simulink model "ChildApp"  (R2023a)
settings: Solver=FixedStepAuto  StartTime=0.0  StopTime=10  RelTol=1e-3
libraries: androidcommunicationlib x6, androiduilib x5, androidaudiovideolib x4, androidsensorlib x3
settings Model: Creator=Hitesh  LastModifiedBy=Hitesh
settings DataIOCC: SaveFormat=Array  InspectSignalLogs=on
settings OptimizationCC: EnhancedBackFolding=on  PassReuseOutputArgsAs=Individual arguments  ZeroExternalMemoryAtStartup=off  ZeroInternalMemoryAtStartup=off  MaxStackSize=64  OptimizeBlockOrder=speed  DifferentSizesBufferReuse=on  OptimizationCustomize=off  EfficientTunableParamExpr=on
settings DebuggingCC: ParameterTunabilityLossMsg=error
settings HardwareCC: ProdBitPerLong=64  ProdLargestAtomicInteger=LongLong  ProdLargestAtomicFloat=Double  ProdLongLongMode=on  ProdHWDeviceType=ARM Compatible->ARM 64-bit (LP64)
settings SFSimCC: MATLABDynamicMemAlloc=off
settings RTWCC: Description=Embedded Coder  SystemTargetFile=ert.tlc  HardwareBoard=Android Device (64bit)  TLCOptions="-aInlineSetEventsForThisBaseRateFcn=TLC_FALSE -aSuppressMultiTaskScheduler=TLC_FALSE  -aRateBasedStepFcn=0"  TemplateMakefile=ert_default_tmf  RTWVerbose=off  Toolchain=Android SDK/NDK Tools
settings CodeAppCC: ForceParamTrailComments=on  IgnoreCustomStorageClasses=off  OperatorAnnotations=on  SimulinkDataObjDesc=on  SFDataObjDesc=on  InsertBlockDesc=on

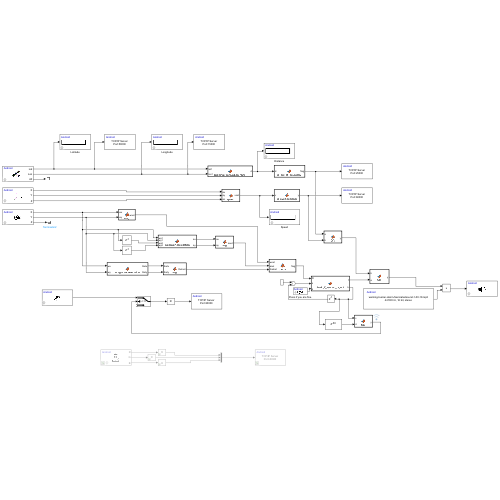
[thumbnail: Simulink's stored preview of the top-level diagram]
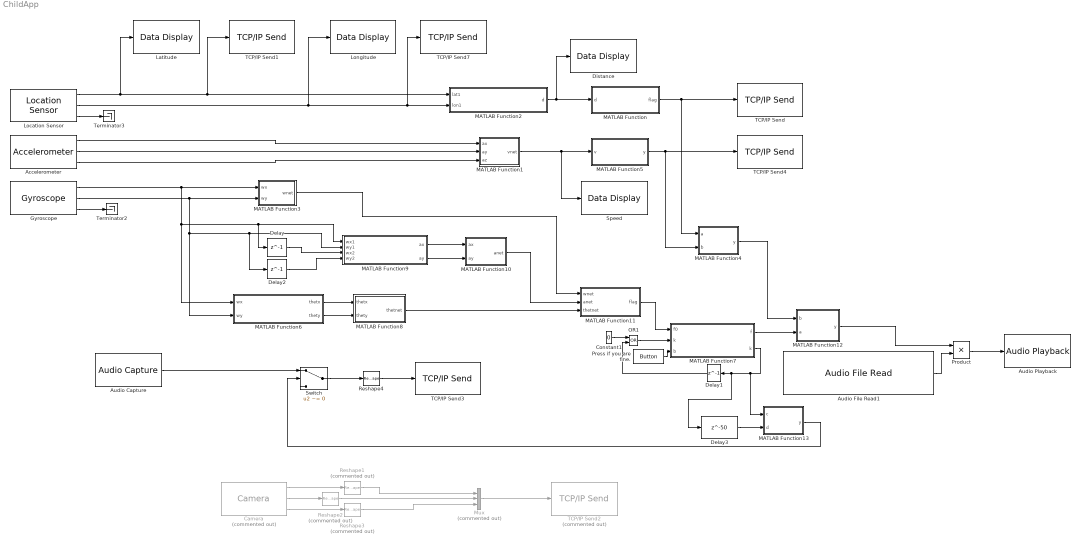
== system ChildApp ==
  Accelerometer : androidsensorlib/Accelerometer  OutputVector=off  SampleTime=0.2  BlockPlatform=Android
  Audio Capture : androidaudiovideolib/Audio Capture  SampleFreq=44100  FrameSize=4410  SampleTime=0.1  SimulateUsing=Code generation  DeviceStr=0  QueueDuration=0  BlockPlatform=Android  AudioSamplingFreq=44100
  Audio File Read1 : androidaudiovideolib/Audio File Read  FileName=C:\Users\Hitesh\Downloads\warning-buzzer-alarm-fascinatedsound-1-00-18.mp3  FrameSize=4410
  Audio Playback : androidaudiovideolib/Audio Playback  SampleFreq=44100  AudioSamplingFreq=44100  SampleTime=0.1  DeviceStr=0  QueueDuration=0  BlockPlatform=Android
  Camera : androidaudiovideolib/Camera  Commented=on  CameraLocation=Back  CameraResolutions=Back - 320x240  Width=320  Height=240  SampleTime=2  BlockPlatform=Android
  Constant1 : Constant  Value=0  OutDataTypeStr=double
  Delay : Delay  DelayLength=1
  Delay1 : Delay  DelayLength=1  InitialCondition=0
  Delay2 : Delay  DelayLength=1
  Delay3 : Delay  DelayLength=50  InitialCondition=0
  Distance : androiduilib/Data Display  DataDisplayId=ChildApp/Distance  Format=Float  Precision=6  SimulateUsing=Code generation  blockPlatform=Android
  Gyroscope : androidsensorlib/Gyroscope  OutputVector=off  SampleTime=0.2  BlockPlatform=Android
  Latitude : androiduilib/Data Display  DataDisplayId=ChildApp/Latitude  Format=Float  Precision=6  SimulateUsing=Code generation  blockPlatform=Android
  Location Sensor : androidsensorlib/Location Sensor  OutputVector=off  SampleTime=0.1  BlockPlatform=Android
  Longitude : androiduilib/Data Display  DataDisplayId=ChildApp/Longitude  Format=Float  Precision=6  SimulateUsing=Code generation  blockPlatform=Android
  MATLAB Function : MATLAB Function  TreatAsAtomicUnit=on
  MATLAB Function1 : MATLAB Function  TreatAsAtomicUnit=on
  MATLAB Function10 : MATLAB Function  TreatAsAtomicUnit=on
  MATLAB Function11 : MATLAB Function  TreatAsAtomicUnit=on
  MATLAB Function12 : MATLAB Function  TreatAsAtomicUnit=on
  MATLAB Function13 : MATLAB Function  TreatAsAtomicUnit=on
  MATLAB Function2 : MATLAB Function  TreatAsAtomicUnit=on
  MATLAB Function3 : MATLAB Function  TreatAsAtomicUnit=on
  MATLAB Function4 : MATLAB Function  TreatAsAtomicUnit=on
  MATLAB Function5 : MATLAB Function  TreatAsAtomicUnit=on
  MATLAB Function6 : MATLAB Function  TreatAsAtomicUnit=on
  MATLAB Function7 : MATLAB Function  TreatAsAtomicUnit=on
  MATLAB Function8 : MATLAB Function  TreatAsAtomicUnit=on
  MATLAB Function9 : MATLAB Function  TreatAsAtomicUnit=on
  Mux : Mux  Commented=on  Inputs=3
  OR1 : Logic  Operator=OR  IconShape=distinctive  AllPortsSameDT=off  OutDataTypeStr=boolean
  Press if you are fine. : androiduilib/Button  ButtonState=Not pressed  ButtonId=ChildApp/Press_if_you_are_fine.  State=off  SampleTime=0.1  BlockPlatform=Android
  Product : Product  InputSameDT=on  OutDataTypeStr=Inherit: Same as first input
  Reshape1 : Reshape  Commented=on  OutputDimensionality=Customize  OutputDimensions=[320*240,1]
  Reshape2 : Reshape  Commented=on  OutputDimensionality=Customize  OutputDimensions=[320*240,1]
  Reshape3 : Reshape  Commented=on  OutputDimensionality=Customize  OutputDimensions=[320*240,1]
  Reshape4 : Reshape  OutputDimensionality=Customize  OutputDimensions=[8820,1]
  Speed : androiduilib/Data Display  DataDisplayId=ChildApp/Speed  Format=Float  Precision=6  SimulateUsing=Code generation  blockPlatform=Android
  Switch : Switch  Criteria=u2 ~= 0  OutDataTypeStr=int16  SaturateOnIntegerOverflow=off  InputSameDT=off
  TCP/IP Send : androidcommunicationlib/TCP//IP Send  TCPSendId=ChildApp/TCP//IP_Send  Mode_=Server  LocalServerPort_=25000  RemoteAddr_=137.158.24.15  RemoteServerPort_=38000  ClientPortBindingSelection_=off  ClientPortToBind_=35000  BlockingMode_=off  BlockTimeout_=0.1
  TCP/IP Send1 : androidcommunicationlib/TCP//IP Send  TCPSendId=ChildApp/TCP//IP_Send1  Mode_=Server  LocalServerPort_=50000  RemoteAddr_=127.0.0.1  RemoteServerPort_=25000  ClientPortBindingSelection_=off  ClientPortToBind_=35000  BlockingMode_=off  BlockTimeout_=0.1
  TCP/IP Send2 : androidcommunicationlib/TCP//IP Send  Commented=on  TCPSendId=ChildApp/TCP//IP_Send2  Mode_=Server  LocalServerPort_=45000  RemoteAddr_=137.158.24.15  RemoteServerPort_=38000  ClientPortBindingSelection_=off  ClientPortToBind_=35000  BlockingMode_=off  BlockTimeout_=0.1
  TCP/IP Send3 : androidcommunicationlib/TCP//IP Send  TCPSendId=ChildApp/TCP//IP_Send3  Mode_=Server  LocalServerPort_=20000  RemoteAddr_=137.158.24.15  RemoteServerPort_=38000  ClientPortBindingSelection_=off  ClientPortToBind_=35000  BlockingMode_=off  BlockTimeout_=0.1
  TCP/IP Send4 : androidcommunicationlib/TCP//IP Send  TCPSendId=ChildApp/TCP//IP_Send4  Mode_=Server  LocalServerPort_=60000  RemoteAddr_=137.158.24.15  RemoteServerPort_=38000  ClientPortBindingSelection_=off  ClientPortToBind_=35000  BlockingMode_=off  BlockTimeout_=0.1
  TCP/IP Send7 : androidcommunicationlib/TCP//IP Send  TCPSendId=ChildApp/TCP//IP_Send7  Mode_=Server  LocalServerPort_=15000  RemoteAddr_=127.0.0.1  RemoteServerPort_=25000  ClientPortBindingSelection_=off  ClientPortToBind_=35000  BlockingMode_=off  BlockTimeout_=0.1
  Terminator2 : Terminator
  Terminator3 : Terminator
  wires:
  Gyroscope/1 -> MATLAB Function6/1(wx), Delay/1, MATLAB Function9/1(wx1), MATLAB Function3/1(wx)
  Gyroscope/2 -> MATLAB Function6/2(wy), Delay2/1, MATLAB Function9/2(wy1), MATLAB Function3/2(wy)
  Delay2/1 -> MATLAB Function9/4(wy2)
  Product/1 -> Audio Playback/1
  MATLAB Function3/1(wnet) -> MATLAB Function11/1(wnet)
  Delay1/1 -> OR1/2
  Delay/1 -> MATLAB Function9/3(wx2)
  MATLAB Function6/1(thetx) -> MATLAB Function8/1(thetx)
  MATLAB Function6/2(thety) -> MATLAB Function8/2(thety)
  Location Sensor/2 -> MATLAB Function2/2(lon1), TCP/IP Send7/1, Longitude/1
  Accelerometer/1 -> MATLAB Function1/1(ax)
  Accelerometer/2 -> MATLAB Function1/2(ay)
  MATLAB Function5/1(y) -> MATLAB Function4/2(b), TCP/IP Send4/1
  Accelerometer/3 -> MATLAB Function1/3(az)
  MATLAB Function9/2(ay) -> MATLAB Function10/2(ay)
  MATLAB Function9/1(ax) -> MATLAB Function10/1(ax)
  MATLAB Function8/1(thetnet) -> MATLAB Function11/3(thetnet)
  Constant1/1 -> OR1/1
  MATLAB Function2/1(d) -> MATLAB Function/1(d), Distance/1
  MATLAB Function11/1(flag) -> MATLAB Function7/1(f0)
  MATLAB Function1/1(vnet) -> Speed/1, MATLAB Function5/1(v)
  MATLAB Function10/1(anet) -> MATLAB Function11/2(anet)
  Press if you are fine./1 -> MATLAB Function7/3(b)
  OR1/1 -> MATLAB Function7/2("k ")
  MATLAB Function7/1(f) -> MATLAB Function12/2(a)
  MATLAB Function/1(flag) -> MATLAB Function4/1(a), TCP/IP Send/1
  MATLAB Function4/1(y) -> MATLAB Function12/1(b)
  MATLAB Function12/1(y) -> Product/1
  Audio File Read1/1 -> Product/2
  Gyroscope/3 -> Terminator2/1
  Location Sensor/3 -> Terminator3/1
  Audio Capture/1 -> Switch/1
  Switch/1 -> Reshape4/1
  Camera/1 -> Reshape1/1
  Camera/3 -> Reshape3/1
  Camera/2 -> Reshape2/1
  Reshape4/1 -> TCP/IP Send3/1
  Mux/1 -> TCP/IP Send2/1
  Reshape1/1 -> Mux/1
  Reshape2/1 -> Mux/2
  Reshape3/1 -> Mux/3
  Delay3/1 -> MATLAB Function13/2(d)
  MATLAB Function13/1(y) -> Switch/2
  MATLAB Function7/2(k) -> MATLAB Function13/1(c), Delay3/1, Delay1/1
  Location Sensor/1 -> MATLAB Function2/1(lat1), TCP/IP Send1/1, Latitude/1

== matlab function ChildApp/MATLAB Function8 ==
  data: thetx input; thetnet output; thety input
function thetnet = mag(thetx,thety)
    thetnet = sqrt(thetx^2+thety^2);
end

== matlab function ChildApp/MATLAB Function9 ==
  data: wx1 input; ax output; wy1 input; wx2 input; wy2 input; ay output
function [ax,ay] = integrateAcceleration(wx1,wy1,wx2,wy2)
    dt=0.2;
    ax=(wx2-wx1)/dt;
    ay=(wy2-wy1)/dt;
end

== matlab function ChildApp/MATLAB Function12 ==
  data: b input; y output; a input
function y = OR(b,a)
    if(b == 1 || a == 1)
        y = int16(1);
    else
        y = int16(0);
    end
end

== matlab function ChildApp/MATLAB Function13 ==
  data: c input; d input; y output
function y = fcn(c,d)
    if(c == 1)
        if(d == 1)
            y = int16(1);
        else
            y = int16(0);
        end
    else
        y = int16(0);
    end
end

== matlab function ChildApp/MATLAB Function1 ==
  data: ax input; vnet output; ay input; az input
function vnet = speed(ax,ay,az)
    dt = 0.2;
    vx = double(ax)*dt;
    vy = double(ay)*dt;
    vz = double(az-9.81)*dt;
    vnet = sqrt(vx^2+vy^2+vz^2);
    if( vnet<= 0.2)
        vnet = 0;
    end
end

== matlab function ChildApp/MATLAB Function2 ==
  data: lat1 input; d output; lon1 input
function d = DistanceFromLatLonInKm(lat1,lon1)
    R = 6371;
    lat2 = 23.2096737;
    lon2 = 72.6836191;
    % Haversine formula
    dlat = deg2rad(lat2-lat1);
    dlon = deg2rad(lon2-lon1); 
    a = sin(dlat/2)^2 + cos(lat1)* cos(lat2) * sin(dlon/2)^2;
    c = 2 * asin(sqrt(complex(a)));  
    d = R * c; % in km
end

== matlab function ChildApp/MATLAB Function ==
  data: d input; flag output
function flag = is_out_of_boundary(d)
    if(d > 0.1)
        flag = int16(1);
    else 
        flag = int16(0);
    end
end

== matlab function ChildApp/MATLAB Function10 ==
  data: ax input; anet output; ay input
function anet = mag(ax,ay)
    anet = sqrt(ax^2+ay^2);
end

== matlab function ChildApp/MATLAB Function4 ==
  data: a input; y output; b input
function y = OR(a,b)
    if(a == 1 || b == 1)
        y = int16(1);
    else 
        y = int16(0);
    end
end

== matlab function ChildApp/MATLAB Function5 ==
  data: v input; y output
function y = is_overspeeding(v)
    if(v>5)
        y = int16(1);
    else
        y = int16(0);
    end

end

== matlab function ChildApp/MATLAB Function11 ==
  data: wnet input; flag output; anet input; thetnet input
function flag = check(wnet,anet,thetnet)
    flag=int16(0);
    if(wnet > 5)
        if(anet > 30 && thetnet > 0.8)
            flag=int16(1);          
        end
    end
end

== matlab function ChildApp/MATLAB Function3 ==
  data: wx input single; wnet output single; wy input single
function wnet = mag(wx,wy)
    wnet = sqrt(wx^2+wy^2);
end

== matlab function ChildApp/MATLAB Function6 ==
  data: wx input; thetx output; wy input; thety output
function [thetx,thety] = integrateAcceleration(wx,wy)
    dt=0.2;
    thetx =double(wx) * dt;
    thety =double(wy) * dt;
end

== matlab function ChildApp/MATLAB Function7 ==
  data: f0 input; f output; k input; k output; b input
function [f,k]= check_if_injured_or_not(f0,k,b)
    if(b == false)
        if(k == false)
            if(f0 == 1)
                k = true;
                f = int16(1);
                return;
            end
            f = int16(0);
        elseif(k == true)
            f = int16(1);
        else
            f = int16(0);
        end
    else
        f = int16(0);
        k = false;
    end
end
